simulink model "ap_12B_cocoSim_pp"  (Simulink 8.5)
settings: Solver=ode3  StartTime=0.0  StopTime=100  FixedStep=Ts  RelTol=1e-3
undefined symbols (not defined in the file): beaver_b, beaver_c, beaver_mass, beaver_S, Cl0, Cl_alpha2_dpt, Cl_beta, Cl_da, Cl_da_alpha, Cl_dr, Cl_p, Cl_r, Cm0, Cm_alpha, Cm_alpha2, Cm_beta2, Cm_de, Cm_df, Cm_dpt, Cm_q, Cm_r, Cn0, Cn_beta, Cn_beta3, Cn_da, Cn_dpt3, Cn_dr, Cn_p, Cn_q, Cn_r, Cx0, Cx_alpha, Cx_alpha2, Cx_alpha3, Cx_df, Cx_df_alpha, Cx_dpt, Cx_dpt2_alpha, Cx_dr, Cx_q, Cy0, Cy_beta, Cy_da, Cy_dr, Cy_dr_alpha, Cy_p, Cy_r, Cz0, Cz_alpha, Cz_alpha3, Cz_de, Cz_de_beta, Cz_df, Cz_df_alpha, Cz_dpt, Cz_q, d2r, fin_act_1, fin_act_2, fin_act_3 ... (+23)
libraries: simulink x12, aerolibtransform2 x9, aerolibutil x7, aerolibasang x7, aerolibadynsys x3, aerolib6dofsys x2, aerolib6dof2 x1
(part 1 of 3)
settings Model: Creator=elliocm  LastModifiedBy=Teme
settings DataIOCC: SignalLoggingSaveFormat=Dataset
settings DebuggingCC: SolverPrmCheckMsg=warning  FcnCallInpInsideContextMsg=EnableAllAsError
settings GRTTargetCC: CombineOutputUpdateFcns=on  GRTInterface=off

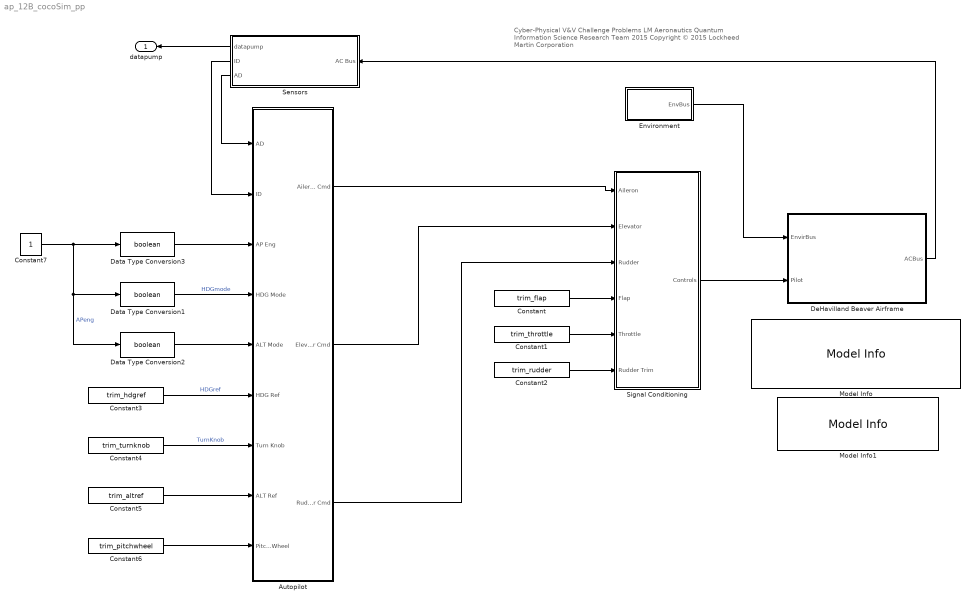
== system ap_12B_cocoSim_pp ==
  note: Cyber-Physical V&V Challenge Problems
      | LM Aeronautics Quantum Information Science Research Team 2015
      | Copyright © 2015 Lockheed Martin Corporation
  Autopilot : Subsystem
  Constant : Constant  Value=trim_flap
  Constant1 : Constant  Value=trim_throttle
  Constant2 : Constant  Value=trim_rudder
  Constant3 : Constant  Value=trim_hdgref
  Constant4 : Constant  Value=trim_turnknob
  Constant5 : Constant  Value=trim_altref
  Constant6 : Constant  Value=trim_pitchwheel
  Constant7 : Constant
  Data Type Conversion1 : DataTypeConversion  OutDataTypeStr=boolean
  Data Type Conversion2 : DataTypeConversion  OutDataTypeStr=boolean
  Data Type Conversion3 : DataTypeConversion  OutDataTypeStr=boolean
  DeHavilland Beaver Airframe : Subsystem
      mask Display: image(imread('asbbeaver.jpg'))
  Environment : Subsystem
  Model Info : simulink/Model-Wide Utilities/Model Info  BlockCM=None  Frame=on  DisplayStringWithTags=|  HorizontalTextAlignment=Center  LeftAlignmentValue=0.5  SourceBlockDiagram=ap_12B_cocoSim_pp  TagMaxNumber=20
      | DeHavilland Beaver model 
      | originally based on work created by
      | Marc Rauw for Delft University of Technology,  
      | http://www.dutchroll.com
      | and subsequently modified by the Mathworks
      | http://www.mathworks.com/matlabcentral/fileexchange/
  Model Info1 : simulink/Model-Wide Utilities/Model Info  BlockCM=None  Frame=on  DisplayStringWithTags=|  HorizontalTextAlignment=Left  LeftAlignmentValue=0.02  SourceBlockDiagram=ap_12B_cocoSim_pp  TagMaxNumber=20
      | FLIGHT CONTROL Demonstration
      | Author: %<LastModifiedBy>
      | Model Version: %<ModelVersion>
      | Date: %<LastModificationDate>
  Sensors : Subsystem
  Signal Conditioning : Subsystem
  datapump : Outport
  wires:
  Constant7/1 -> Data Type Conversion2/1, Data Type Conversion1/1, Data Type Conversion3/1  "APeng"
  Data Type Conversion1/1 -> Autopilot/4(HDG Mode)  "HDGmode"
  Data Type Conversion2/1 -> Autopilot/5(ALT Mode)
  Constant3/1 -> Autopilot/6(HDG Ref)  "HDGref"
  Constant4/1 -> Autopilot/7(Turn Knob)  "TurnKnob"
  Constant5/1 -> Autopilot/8(ALT Ref)
  Constant6/1 -> Autopilot/9(Pitch Wheel)
  Autopilot/1(Aileron Cmd) -> Signal Conditioning/1(Aileron)
  Autopilot/2(Elevator Cmd) -> Signal Conditioning/2(Elevator)
  Autopilot/3(Rudder Cmd) -> Signal Conditioning/3(Rudder)
  DeHavilland Beaver Airframe/1(ACBus) -> Sensors/1(AC Bus)
  Constant/1 -> Signal Conditioning/4(Flap)
  Constant1/1 -> Signal Conditioning/5(Throttle)
  Constant2/1 -> Signal Conditioning/6(Rudder Trim)
  Signal Conditioning/1(Controls) -> DeHavilland Beaver Airframe/2(Pilot)
  Environment/1(EnvBus) -> DeHavilland Beaver Airframe/1(EnvirBus)
  Sensors/3(AD) -> Autopilot/1(AD)
  Sensors/2(ID) -> Autopilot/2(ID)
  Data Type Conversion3/1 -> Autopilot/3(AP Eng)
  Sensors/1(datapump) -> datapump/1

== system ap_12B_cocoSim_pp/Autopilot ==
  note: Autopilot
  AD : Inport
  ID : Inport  Port=2
  AP Eng : Inport  Port=3  OutMin=0  OutMax=1  OutDataTypeStr=boolean  PortDimensions=1
  HDG Mode : Inport  Port=4  OutMin=0  OutMax=1  OutDataTypeStr=boolean  PortDimensions=1
  ALT Mode : Inport  Port=5  OutMin=0  OutMax=1  OutDataTypeStr=boolean  PortDimensions=1
  HDG Ref : Inport  Port=6  OutMin=-180  OutMax=180  OutDataTypeStr=double  PortDimensions=1
  Turn Knob : Inport  Port=7  OutMin=-45  OutMax=45  OutDataTypeStr=double  PortDimensions=1
  ALT Ref : Inport  Port=8  OutMin=0  OutMax=65000  OutDataTypeStr=double  PortDimensions=1
  Pitch Wheel : Inport  Port=9  OutMin=-30  OutMax=30  OutDataTypeStr=double  PortDimensions=1
  Bus Selector : BusSelector  OutputSignals=phi,psi,p,theta,q,r
  Bus Selector1 : BusSelector  OutputSignals=alt,altRate,airspeed
  Model Info : simulink/Model-Wide Utilities/Model Info  BlockCM=None  Frame=on  DisplayStringWithTags=|  HorizontalTextAlignment=Left  LeftAlignmentValue=0.02  SourceBlockDiagram=ap_12B_cocoSim_pp  TagMaxNumber=20
      | Autopilot
      | Author: %<LastModifiedBy>
      | Date: %<LastModificationDate>
      | Model Version: %<ModelVersion>
  Pitch_Autopilot : Subsystem
  Roll_Autopilot : Subsystem
  Yaw_damper : Subsystem
  Aileron Cmd : Outport  OutDataTypeStr=double  PortDimensions=1  SampleTime=[0.025000000000000001,0]
  Elevator Cmd : Outport  Port=2  OutDataTypeStr=double  PortDimensions=1  SampleTime=[0.025000000000000001,0]
  Rudder Cmd : Outport  Port=3  OutDataTypeStr=double  PortDimensions=1  SampleTime=[0.025000000000000001,0]
  wires:
  Roll_Autopilot/1(Ail Cmd) -> Aileron Cmd/1
  HDG Ref/1 -> Roll_Autopilot/7(HDG Ref)
  Bus Selector/6 -> Yaw_damper/2(R), Pitch_Autopilot/4(R)  "<r>"
  Bus Selector1/3 -> Yaw_damper/3(TAS), Roll_Autopilot/4(TAS), Pitch_Autopilot/7(TAS)  "<airspeed>"
  HDG Mode/1 -> Roll_Autopilot/6(HDG Mode)
  Pitch_Autopilot/1(Elv Cmd) -> Elevator Cmd/1
  ALT Mode/1 -> Pitch_Autopilot/9(ALT Mode)
  ALT Ref/1 -> Pitch_Autopilot/10(Alt Ref)
  Pitch Wheel/1 -> Pitch_Autopilot/11("Pitch Wheel ")
  Bus Selector1/1 -> Pitch_Autopilot/5(Alt)  "<alt>"
  Yaw_damper/1(Rud Cmd) -> Rudder Cmd/1
  AP Eng/1 -> Yaw_damper/4(AP Eng), Roll_Autopilot/5(AP Eng), Pitch_Autopilot/8(AP Eng1)
  Bus Selector/3 -> Roll_Autopilot/3(p)  "<p>"
  Turn Knob/1 -> Roll_Autopilot/8(Turn Knob)
  Bus Selector/1 -> Pitch_Autopilot/1(Phi), Yaw_damper/1(Phi), Roll_Autopilot/1(Phi)  "<phi>"
  Bus Selector/2 -> Roll_Autopilot/2(Psi)  "<psi>"
  Bus Selector/5 -> Pitch_Autopilot/3(Q)  "<q>"
  Bus Selector/4 -> Pitch_Autopilot/2(Theta)  "<theta>"
  ID/1 -> Bus Selector/1
  AD/1 -> Bus Selector1/1
  Bus Selector1/2 -> Pitch_Autopilot/6(Alt Rate)  "<altRate>"

== system ap_12B_cocoSim_pp/DeHavilland Beaver Airframe ==
  note: DeHavilland Beaver Airframe
  EnvirBus : Inport
  Pilot : Inport  Port=2
  Aircraft Dynamics : Subsystem
  Calculate Parameters : Subsystem
  ACBus : Outport
  wires:
  Pilot/1 -> Aircraft Dynamics/1(Pilot)
  Aircraft Dynamics/1(AC Bus) -> ACBus/1, Calculate Parameters/2(ACBus)
  EnvirBus/1 -> Aircraft Dynamics/2(EnvirBus), Calculate Parameters/1(EnvirBus)
  Calculate Parameters/1(FltParams) -> Aircraft Dynamics/3(FltParams)

== system ap_12B_cocoSim_pp/Environment ==
  note: Environment
  Bus Creator : BusCreator  Inputs=3
  Bus Creator1 : BusCreator  Inputs=2
  Mux : Mux  Inputs=3
  Mux1 : Mux  Inputs=3
  g_mps2 : Constant  Value=9.799
  rho_kgpm3 : Constant  Value=0.9862
  wind_mps : Constant  Value=0
  EnvBus : Outport
  wires:
  g_mps2/1 -> Bus Creator/1  "g"
  Mux1/1 -> Bus Creator1/2  "pqr_wind"
  Mux/1 -> Bus Creator1/1  "uvw_wind"
  Bus Creator1/1 -> Bus Creator/3  "Vwind"
  Bus Creator/1 -> EnvBus/1
  rho_kgpm3/1 -> Bus Creator/2  "rho"
  wind_mps/1 -> Mux1/3, Mux1/2, Mux1/1, Mux/3, Mux/2, Mux/1

== system ap_12B_cocoSim_pp/Sensors ==
  AC Bus : Inport
  Air Data Sensor : Subsystem
  Bus Creator : BusCreator  Inputs=6
  Bus Creator1 : BusCreator  Inputs=5
  Bus Creator2 : BusCreator  Inputs=2
  Display : Display
  Display1 : Display
  Inertial Data Sensor : Subsystem
  Scope : Scope  NumInputPorts=5
      settings: YMin=-125~-3.5~-1.75~65~2000  YMax=125~3.5~1.75~150~7500  SaveName=ScopeData11
  Scope1 : Scope  NumInputPorts=6
      settings: YMin=-5~-5~-5~-5~-5~-5  YMax=5~5~5~5~5~5  SaveName=ScopeData12
  datapump : Outport
  ID : Outport  Port=2
  AD : Outport  Port=3
  wires:
  AC Bus/1 -> Air Data Sensor/1(AC Bus), Inertial Data Sensor/1(AC Bus)
  Inertial Data Sensor/3(psi) -> Scope1/3, Bus Creator/3  "psi"
  Inertial Data Sensor/2(theta) -> Scope1/2, Bus Creator/2  "theta"
  Inertial Data Sensor/4(p) -> Scope1/4, Bus Creator/4  "p"
  Inertial Data Sensor/1(phi) -> Scope1/1, Bus Creator/1
  Inertial Data Sensor/5(q) -> Scope1/5, Bus Creator/5  "q"
  Inertial Data Sensor/6(r) -> Scope1/6, Bus Creator/6  "r"
  Bus Creator/1 -> Bus Creator2/1, Display/1, ID/1  "ID"
  Air Data Sensor/1(altRate) -> Scope/1, Bus Creator1/1  "altRate"
  Air Data Sensor/2(alpha) -> Scope/2, Bus Creator1/2  "alpha"
  Air Data Sensor/3(beta) -> Scope/3, Bus Creator1/3  "beta"
  Air Data Sensor/4(airspeed) -> Scope/4, Bus Creator1/4  "airspeed"
  Air Data Sensor/5(alt) -> Scope/5, Bus Creator1/5  "alt"
  Bus Creator1/1 -> Bus Creator2/2, Display1/1, AD/1  "AD"
  Bus Creator2/1 -> datapump/1

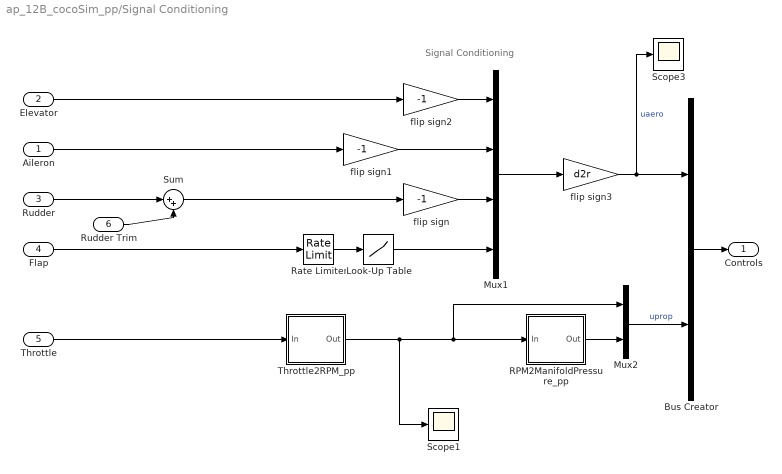
== system ap_12B_cocoSim_pp/Signal Conditioning ==
  note: Signal Conditioning
  Aileron : Inport
  Elevator : Inport  Port=2
  Rudder : Inport  Port=3
  Flap : Inport  Port=4
  Throttle : Inport  Port=5
  Rudder Trim : Inport  Port=6
  Bus Creator : BusCreator  Inputs=2
  Look-Up Table : Lookup  InputValues=[0:3]  Table=[0 4 10 20]  SaturateOnIntegerOverflow=on
  Mux1 : Mux
  Mux2 : Mux  Inputs=2
  RPM2ManifoldPressure_pp : Subsystem  TreatAsAtomicUnit=on
  Rate Limiter : RateLimiter  RisingSlewLimit=0.5  FallingSlewLimit=-0.5
  Scope1 : Scope
      settings: SaveName=ScopeData7
  Scope3 : Scope
      settings: SaveName=ScopeData6
  Sum : Sum  Inputs=|++
  Throttle2RPM_pp : Subsystem  TreatAsAtomicUnit=on
  flip sign : Gain  Gain=-1  SaturateOnIntegerOverflow=on  OutDataTypeStr=Inherit: Same as input  ParamDataTypeStr=Inherit: Same as input
  flip sign1 : Gain  Gain=-1  SaturateOnIntegerOverflow=on  OutDataTypeStr=Inherit: Same as input  ParamDataTypeStr=Inherit: Same as input
  flip sign2 : Gain  Gain=-1  SaturateOnIntegerOverflow=on  OutDataTypeStr=Inherit: Same as input  ParamDataTypeStr=Inherit: Same as input
  flip sign3 : Gain  Gain=d2r  SaturateOnIntegerOverflow=on  OutDataTypeStr=Inherit: Same as input  ParamDataTypeStr=Inherit: Same as input
  Controls : Outport
  wires:
  Bus Creator/1 -> Controls/1
  Throttle/1 -> Throttle2RPM_pp/1(In)
  Sum/1 -> flip sign/1
  Aileron/1 -> flip sign1/1
  Elevator/1 -> flip sign2/1
  flip sign2/1 -> Mux1/1
  flip sign1/1 -> Mux1/2
  Throttle2RPM_pp/1(Out) -> Scope1/1, RPM2ManifoldPressure_pp/1(In), Mux2/1
  flip sign/1 -> Mux1/3
  Mux2/1 -> Bus Creator/2  "uprop"
  RPM2ManifoldPressure_pp/1(Out) -> Mux2/2
  flip sign3/1 -> Scope3/1, Bus Creator/1  "uaero"
  Mux1/1 -> flip sign3/1
  Look-Up Table/1 -> Mux1/4
  Rate Limiter/1 -> Look-Up Table/1
  Rudder/1 -> Sum/1
  Rudder Trim/1 -> Sum/2
  Flap/1 -> Rate Limiter/1

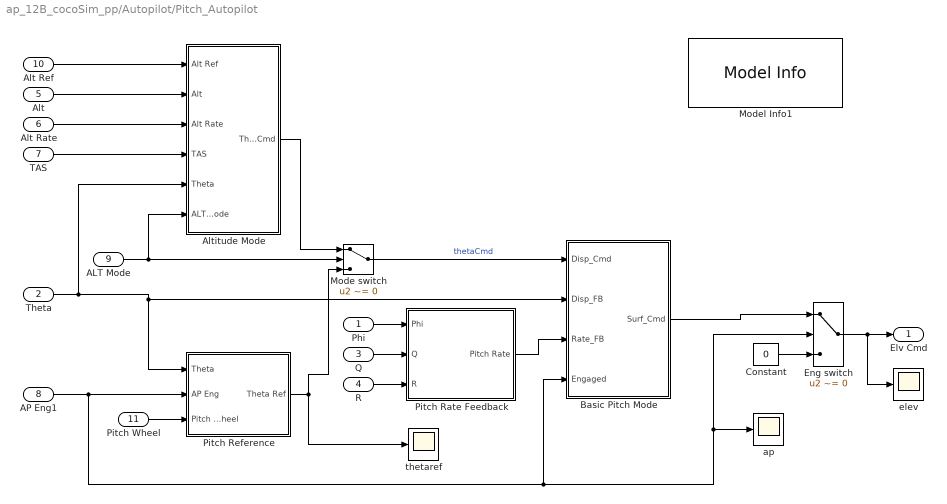
== system ap_12B_cocoSim_pp/Autopilot/Pitch_Autopilot ==
  Phi : Inport  OutDataTypeStr=double  PortDimensions=1  SampleTime=1/40  Interpolate=off
  Theta : Inport  Port=2  OutDataTypeStr=double  PortDimensions=1  SampleTime=1/40  Interpolate=off
  Q : Inport  Port=3  OutDataTypeStr=double  PortDimensions=1  SampleTime=1/40  Interpolate=off
  R : Inport  Port=4  OutDataTypeStr=double  PortDimensions=1  SampleTime=1/40  Interpolate=off
  Alt : Inport  Port=5  OutDataTypeStr=double  PortDimensions=1  SampleTime=1/40  Interpolate=off
  Alt Rate : Inport  Port=6  OutDataTypeStr=double  PortDimensions=1  SampleTime=1/40  Interpolate=off
  TAS : Inport  Port=7  OutDataTypeStr=double  PortDimensions=1  SampleTime=1/40  Interpolate=off
  AP Eng1 : Inport  Port=8  OutDataTypeStr=boolean  PortDimensions=1  SampleTime=1/40  Interpolate=off
  ALT Mode : Inport  Port=9  OutDataTypeStr=boolean  PortDimensions=1  SampleTime=1/40  Interpolate=off
  Alt Ref : Inport  Port=10  OutDataTypeStr=double  PortDimensions=1  SampleTime=1/40  Interpolate=off
  "Pitch Wheel " : Inport  Port=11  OutDataTypeStr=double  PortDimensions=1  SampleTime=1/40  Interpolate=off
  Altitude Mode : Subsystem
  Basic Pitch Mode : Subsystem
  Constant : Constant  Value=0  OutDataTypeStr=double
  Eng switch : Switch  Criteria=u2 ~= 0
  Mode switch : Switch  Criteria=u2 ~= 0
  Model Info1 : simulink/Model-Wide Utilities/Model Info  BlockCM=None  Frame=on  DisplayStringWithTags=|  HorizontalTextAlignment=Left  LeftAlignmentValue=0.02  SourceBlockDiagram=ap_12B_cocoSim_pp  TagMaxNumber=20
      | Pitch Autopilot
      | Author: %<LastModifiedBy>
      | Date: %<LastModificationDate>
      | Model Version: %<ModelVersion>
  Pitch Rate Feedback : Subsystem  TreatAsAtomicUnit=on
      settings: RTWSystemCode=Inline
  Pitch Reference : Subsystem  TreatAsAtomicUnit=on
      settings: RTWSystemCode=Inline
  ap : Scope
      settings: SaveName=ScopeData29
  elev : Scope
      settings: SaveName=ScopeData33
  thetaref : Scope
      settings: SaveName=ScopeData37
  Elv Cmd : Outport  OutDataTypeStr=double  PortDimensions=1  SampleTime=1/40
  wires:
  "Pitch Wheel "/1 -> Pitch Reference/3(Pitch Wheel)
  Pitch Rate Feedback/1(Pitch Rate) -> Basic Pitch Mode/3(Rate_FB)
  Alt Ref/1 -> Altitude Mode/1(Alt Ref)
  Theta/1 -> Altitude Mode/5(Theta), Pitch Reference/1(Theta), Basic Pitch Mode/2("Disp_FB ")
  Q/1 -> Pitch Rate Feedback/2(Q)
  Eng switch/1 -> elev/1, Elv Cmd/1
  Constant/1 -> Eng switch/3
  Phi/1 -> Pitch Rate Feedback/1(Phi)
  R/1 -> Pitch Rate Feedback/3(R)
  TAS/1 -> Altitude Mode/4(TAS)
  Pitch Reference/1(Theta Ref) -> thetaref/1, Mode switch/3
  Alt/1 -> Altitude Mode/2(Alt)
  Alt Rate/1 -> Altitude Mode/3(Alt Rate)
  Mode switch/1 -> Basic Pitch Mode/1(Disp_Cmd)  "thetaCmd"
  ALT Mode/1 -> Altitude Mode/6(ALT Mode), Mode switch/2
  Altitude Mode/1(Theta Cmd) -> Mode switch/1
  AP Eng1/1 -> Eng switch/2, ap/1, Basic Pitch Mode/4(Engaged), Pitch Reference/2(AP Eng)
  Basic Pitch Mode/1(Surf_Cmd) -> Eng switch/1

== system ap_12B_cocoSim_pp/Autopilot/Roll_Autopilot ==
  Phi : Inport  RequirementInfo={'other' 'do178b_autopilot_requirements.docx' '@Simulink_requirement_item_3' 'true' '1.3. Roll Hold Reference' ' ' ; 'other' 'do178b_autopilot_requirements.docx' '@Simulink_requirement_item_4' 'true' '1.4. Roll Performance' '' } %GIDa_bd230888_8e4f_4651_af95_bb052af88046  OutMin=-180  OutMax=180  OutDataTypeStr=double  PortDimensions=1  SampleTime=1/40  Interpolate=off
  Psi : Inport  RequirementInfo={'other' 'do178b_autopilot_requirements.docx' '@Simulink_requirement_item_10' 'true' '1.10. Heading Performance' '' } %GIDa_dd31966d_985c_45f4_accd_9bdc5dfb2899  Port=2  OutMin=-180  OutMax=180  OutDataTypeStr=double  PortDimensions=1  SampleTime=1/40  Interpolate=off
  p : Inport  RequirementInfo={'other' 'do178b_autopilot_requirements.docx' '@Simulink_requirement_item_4' 'true' '1.4. Roll Performance' '' } %GIDa_df9fbc51_a2ae_43d6_98fc_cabd7d0ca57e  Port=3  OutMin=-180  OutMax=180  OutDataTypeStr=double  PortDimensions=1  Interpolate=off
  TAS : Inport  RequirementInfo={'other' 'do178b_autopilot_requirements.docx' '@Simulink_requirement_item_10' 'true' '1.10. Heading Performance' '' } %GIDa_635b1e96_333c_4ec3_a8eb_fd034fb3c326  Port=4  OutMin=0  OutMax=1000  OutDataTypeStr=double  PortDimensions=1  SampleTime=1/40  Interpolate=off
  AP Eng : Inport  RequirementInfo={'other' 'do178b_autopilot_requirements.docx' '@Simulink_requirement_item_1' 'true' '1.1. Roll Autopilot Engage Control' ' ' ; 'other' 'do178b_autopilot_requirements.docx' '@Simulink_requirement_item_3' 'true' '1.3. Roll Hold Reference' ' ' ; 'other' 'do178b_autopilot_requirements.docx' '@Simulink_requirement_item_4' 'true' '1.4. Roll Performance' '' } %GIDa_32c51ab2_ea73_4f85_bfd4_20a740fc7588  Port=5  OutDataTypeStr=boolean  PortDimensions=1  SampleTime=1/40  Interpolate=off
  HDG Mode : Inport  RequirementInfo={'other' 'do178b_autopilot_requirements.docx' '@Simulink_requirement_item_2' 'true' '1.2. Roll Hold Mode' ' ' ; 'other' 'do178b_autopilot_requirements.docx' '@Simulink_requirement_item_8' 'true' '1.8. Heading Hold Mode' '' } %GIDa_2622cebb_32cd_44ec_b3f0_415d7d3b06da  Port=6  OutDataTypeStr=boolean  PortDimensions=1  SampleTime=1/40  Interpolate=off
  HDG Ref : Inport  RequirementInfo={'other' 'do178b_autopilot_requirements.docx' '@Simulink_requirement_item_9' 'true' '1.9. Heading Hold Reference' ' ' ; 'other' 'do178b_autopilot_requirements.docx' '@Simulink_requirement_item_10' 'true' '1.10. Heading Performance' '' } %GIDa_1720625b_9837_4e8c_b101_844eceaa1bed  Port=7  OutMin=-180  OutMax=180  OutDataTypeStr=double  PortDimensions=1  SampleTime=1/40  Interpolate=off
  Turn Knob : Inport  RequirementInfo={'other' 'do178b_autopilot_requirements.docx' '@Simulink_requirement_item_3' 'true' '1.3. Roll Hold Reference' '' } %GIDa_9853f841_f607_4644_995f_a277bee0f0d4  Port=8  OutMin=-45  OutMax=45  OutDataTypeStr=double  PortDimensions=1  SampleTime=1/40  Interpolate=off
  Basic Roll Mode : Subsystem
  Eng switch : Switch  RequirementInfo={'other' 'do178b_autopilot_requirements.docx' '' 'true' '1.1. Roll Autopilot Engage Control' ' ' } %GIDa_48ca80c0_8a95_4669_9a3a_89e9ba2b13bd  Criteria=u2 ~= 0
  Heading Mode : Subsystem
  Mode switch : Switch  RequirementInfo={'other' 'do178b_autopilot_requirements.docx' '@Simulink_requirement_item_2' 'true' '1.2. Roll Hold Mode' ' ' ; 'other' 'do178b_autopilot_requirements.docx' '@Simulink_requirement_item_4' 'true' '1.4. Roll Performance' ' ' ; 'other' 'do178b_autopilot_requirements.docx' '@Simulink_requirement_item_8' 'true' '1.8. Heading Hold Mode' ' ' ; 'other' 'do178b_autopilot_requirements.docx' '@Simulink_requirement_item_10' 'true' '1.10. Heading Performance' '' } %GIDa_7ff7f3f6_daae_4da2_99fc_89be4661dc9b  Criteria=u2 ~= 0
  Model Info : simulink/Model-Wide Utilities/Model Info  RequirementInfo={} %GIDa_8a06d8a3_adc0_4540_b134_32bcff30f9aa  BlockCM=None  Frame=on  DisplayStringWithTags=|  HorizontalTextAlignment=Left  LeftAlignmentValue=0.02  SourceBlockDiagram=ap_12B_cocoSim_pp  TagMaxNumber=20
      | Roll Autopilot
      | Author: %<LastModifiedBy>
      | Model Version: %<ModelVersion>
      | Date: %<LastModificationDate>
  Roll Reference : Subsystem  RequirementInfo={'other' 'do178b_autopilot_requirements.docx' '@Simulink_requirement_item_3' 'true' '1.3. Roll Hold Reference' '' } %GIDa_54b8aa08_ab27_4ed0_a6e8_f116b5006373  TreatAsAtomicUnit=on
      settings: RTWSystemCode=Inline
  zero : Constant  RequirementInfo={'other' 'do178b_autopilot_requirements.docx' '' 'true' '1.1. Roll Autopilot Engage Control' '' } %GIDa_447f47c4_0c8a_430f_82c0_d7755d441746  Value=0  OutDataTypeStr=double
  Ail Cmd : Outport  RequirementInfo={'other' 'do178b_autopilot_requirements.docx' '' 'true' '1.1. Roll Autopilot Engage Control' ' ' } %GIDa_ea4f82f9_e42f_4b8f_8523_427f9e113761  OutDataTypeStr=double  PortDimensions=1  SampleTime=1/40
  wires:
  HDG Ref/1 -> Heading Mode/1(Psi Ref)
  Heading Mode/1(Phi Cmd) -> Mode switch/1
  Basic Roll Mode/1(Surf_Cmd) -> Eng switch/1
  Mode switch/1 -> Basic Roll Mode/1(Disp_Cmd)  "phiCmd"
  Eng switch/1 -> Ail Cmd/1
  AP Eng/1 -> Roll Reference/2(AP eng), Basic Roll Mode/4(Engaged), Eng switch/2
  TAS/1 -> Heading Mode/3(TAS)
  HDG Mode/1 -> Mode switch/2
  Roll Reference/1(Phi Ref) -> Mode switch/3
  Turn Knob/1 -> Roll Reference/3(Turn Knob)
  zero/1 -> Eng switch/3
  p/1 -> Basic Roll Mode/3(Rate_FB)
  Phi/1 -> Basic Roll Mode/2("Disp_FB "), Roll Reference/1(Phi)
  Psi/1 -> Heading Mode/2(Psi)

== system ap_12B_cocoSim_pp/Autopilot/Yaw_damper ==
  Phi : Inport  OutDataTypeStr=double  PortDimensions=1  SampleTime=1/40  Interpolate=off
  R : Inport  Port=2  OutDataTypeStr=double  PortDimensions=1  SampleTime=1/40  Interpolate=off
  TAS : Inport  Port=3  OutDataTypeStr=double  PortDimensions=1  SampleTime=1/40  Interpolate=off
  AP Eng : Inport  Port=4  OutDataTypeStr=boolean  PortDimensions=1  SampleTime=1/40  Interpolate=off
  Basic Yaw Damper : Subsystem  TreatAsAtomicUnit=on
      settings: RTWSystemCode=Inline
  Constant : Constant  Value=0  OutDataTypeStr=double
  Eng switch : Switch  Criteria=u2 ~= 0
  Model Info1 : simulink/Model-Wide Utilities/Model Info  BlockCM=None  Frame=on  DisplayStringWithTags=|  HorizontalTextAlignment=Left  LeftAlignmentValue=0.02  SourceBlockDiagram=ap_12B_cocoSim_pp  TagMaxNumber=20
      | Yaw Damper
      | Author: %<LastModifiedBy>
      | Version: %<ModelVersion>
      | Date: %<LastModificationDate>
  Rud Cmd : Outport  OutDataTypeStr=double  PortDimensions=1  SampleTime=1/40
  wires:
  Phi/1 -> Basic Yaw Damper/1("Phi ")
  R/1 -> Basic Yaw Damper/2(R)
  Constant/1 -> Eng switch/3
  TAS/1 -> Basic Yaw Damper/3(TAS)
  Basic Yaw Damper/1(Rud Cmd) -> Eng switch/1
  Eng switch/1 -> Rud Cmd/1
  AP Eng/1 -> Eng switch/2

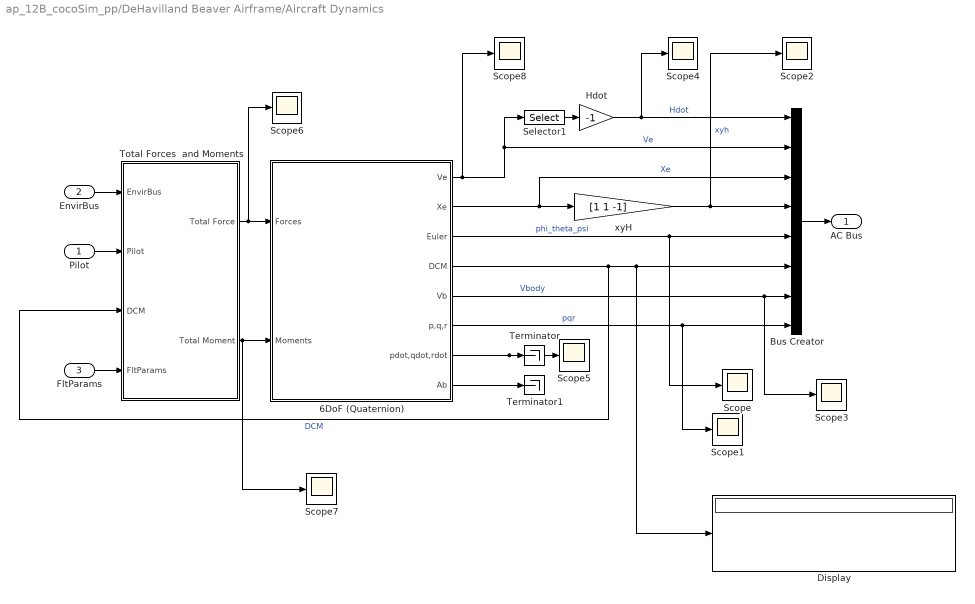
== system ap_12B_cocoSim_pp/DeHavilland Beaver Airframe/Aircraft Dynamics ==
  Pilot : Inport
  EnvirBus : Inport  Port=2
  FltParams : Inport  Port=3
  6DoF (Quaternion) : Subsystem
  Bus Creator : BusCreator  Inputs=8
  Display : Display
  Hdot : Gain  Gain=-1  SaturateOnIntegerOverflow=on  OutDataTypeStr=Inherit: Same as input  ParamDataTypeStr=Inherit: Same as input
  Scope{,1..8} (9 alike) : Scope
      Scope2 settings: SaveName=ScopeData2
      Scope3 settings: SaveName=ScopeData3
      Scope4 settings: SaveName=ScopeData5
      Scope5 settings: SaveName=ScopeData10
      Scope6 settings: SaveName=ScopeData20
      Scope7 settings: SaveName=ScopeData21
      Scope8 settings: SaveName=ScopeData23
  Selector1 : Selector  InputPortWidth=3  Indices=[3]
  Terminator : Terminator
  Terminator1 : Terminator
  Total Forces  and Moments : Subsystem
  xyH : Gain  Gain=[1 1 -1]  SaturateOnIntegerOverflow=on  OutDataTypeStr=Inherit: Same as input  ParamDataTypeStr=Inherit: Same as input
  AC Bus : Outport
  wires:
  6DoF (Quaternion)/4(DCM) -> Display/1, Bus Creator/6, Total Forces  and Moments/3(DCM)  "DCM"
  6DoF (Quaternion)/3(Euler) -> Scope/1, Bus Creator/5  "phi_theta_psi"
  6DoF (Quaternion)/2(Xe) -> xyH/1, Bus Creator/3  "Xe"
  6DoF (Quaternion)/5(Vb) -> Scope3/1, Bus Creator/7  "Vbody"
  6DoF (Quaternion)/7(pdot,qdot,rdot) -> Scope5/1, Terminator/1
  6DoF (Quaternion)/1(Ve) -> Scope8/1, Selector1/1, Bus Creator/2  "Ve"
  Pilot/1 -> Total Forces  and Moments/2(Pilot)
  Selector1/1 -> Hdot/1
  Total Forces  and Moments/1(Total Force) -> Scope6/1, 6DoF (Quaternion)/1(Forces)
  Total Forces  and Moments/2(Total Moment) -> Scope7/1, 6DoF (Quaternion)/2(Moments)
  xyH/1 -> Scope2/1, Bus Creator/4  "xyh"
  Hdot/1 -> Scope4/1, Bus Creator/1  "Hdot"
  6DoF (Quaternion)/8(Ab) -> Terminator1/1
  Bus Creator/1 -> AC Bus/1
  EnvirBus/1 -> Total Forces  and Moments/1(EnvirBus)
  6DoF (Quaternion)/6(p,q,r) -> Scope1/1, Bus Creator/8  "pqr"
  FltParams/1 -> Total Forces  and Moments/4(FltParams)

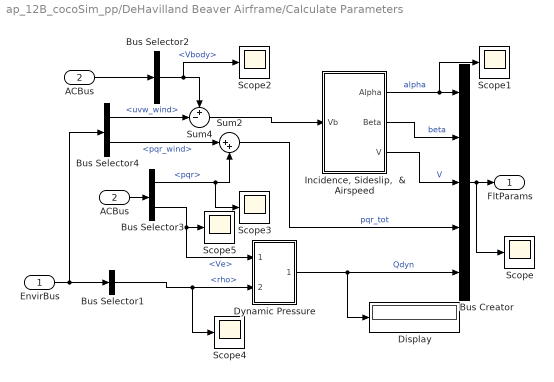
== system ap_12B_cocoSim_pp/DeHavilland Beaver Airframe/Calculate Parameters ==
  EnvirBus : Inport
  ACBus : Inport  Port=2
  " Incidence, Sideslip,  & Airspeed" : Subsystem
  "ACBus " : InportShadow  Port=2
  Bus Creator : BusCreator  Inputs=5
  Bus Selector1 : BusSelector  OutputSignals=rho
  Bus Selector2 : BusSelector  OutputSignals=Vbody
  Bus Selector3 : BusSelector  OutputSignals=pqr,Ve
  Bus Selector4 : BusSelector  OutputSignals=Vwind.uvw_wind,Vwind.pqr_wind
  Display : Display
  Dynamic Pressure : Subsystem
  Scope{,1..5} (6 alike) : Scope
      Scope settings: SaveName=ScopeData14
      Scope1 settings: SaveName=ScopeData15
      Scope2 settings: SaveName=ScopeData16
      Scope3 settings: SaveName=ScopeData17
      Scope4 settings: SaveName=ScopeData18
      Scope5 settings: SaveName=ScopeData19
  Sum2 : Sum  Inputs=|++  SaturateOnIntegerOverflow=on  InputSameDT=on  OutDataTypeStr=Inherit: Same as first input
  Sum4 : Sum  Inputs=+-|  SaturateOnIntegerOverflow=on  InputSameDT=on  OutDataTypeStr=Inherit: Same as first input
  FltParams : Outport
  wires:
  "ACBus "/1 -> Bus Selector2/1
  Bus Creator/1 -> Scope/1, FltParams/1
  Bus Selector3/1 -> Scope3/1, Sum2/2  "<pqr>"
  ACBus/1 -> Bus Selector3/1
  Bus Selector1/1 -> Scope4/1, Dynamic Pressure/2(Air Density)  "<rho>"
  EnvirBus/1 -> Bus Selector1/1, Bus Selector4/1
  Dynamic Pressure/1(qbar) -> Display/1, Bus Creator/5  "Qdyn"
  Bus Selector3/2 -> Scope5/1, Dynamic Pressure/1(Velocity)  "<Ve>"
  Bus Selector4/2 -> Sum2/1  "<pqr_wind>"
  Sum4/1 -> " Incidence, Sideslip,  & Airspeed"/1(Vb)
  " Incidence, Sideslip,  & Airspeed"/1(Alpha) -> Scope1/1, Bus Creator/1  "alpha"
  " Incidence, Sideslip,  & Airspeed"/2(Beta) -> Bus Creator/2  "beta"
  " Incidence, Sideslip,  & Airspeed"/3(V) -> Bus Creator/3  "V"
  Bus Selector2/1 -> Scope2/1, Sum4/1  "<Vbody>"
  Bus Selector4/1 -> Sum4/2  "<uvw_wind>"
  Sum2/1 -> Bus Creator/4  "pqr_tot"

== system ap_12B_cocoSim_pp/Sensors/Air Data Sensor ==
  note: Air Data Sensor
  AC Bus : Inport
  " Incidence, Sideslip,  & Airspeed" : Subsystem
  Bus Selector1 : BusSelector  OutputSignals=Hdot,Vbody,xyh
  Constant1 : Constant  Value=trim_v
  Constant2 : Constant  Value=0.0
  Constant3 : Constant  Value=trim_altref
  Selector1 : Selector  InputPortWidth=3  Indices=[3]
  flip sign1 : Gain  Gain=m2ft  SaturateOnIntegerOverflow=on  OutDataTypeStr=Inherit: Same as input  ParamDataTypeStr=Inherit: Same as input
  flip sign2 : Gain  Gain=m2ft  SaturateOnIntegerOverflow=on  OutDataTypeStr=Inherit: Same as input  ParamDataTypeStr=Inherit: Same as input
  flip sign3 : Gain  Gain=m2ft  SaturateOnIntegerOverflow=on  OutDataTypeStr=Inherit: Same as input  ParamDataTypeStr=Inherit: Same as input
  ic1 : Subsystem
  ic2 : Subsystem
  ic3 : Subsystem
  altRate : Outport
  alpha : Outport  Port=2
  beta : Outport  Port=3
  airspeed : Outport  Port=4
  alt : Outport  Port=5
  wires:
  Bus Selector1/1 -> flip sign2/1  "<Hdot>"
  ic1/1(y) -> flip sign1/1
  ic3/1(y) -> altRate/1  "altRate"
  Bus Selector1/3 -> Selector1/1  "<xyh>"
  flip sign1/1 -> " Incidence, Sideslip,  & Airspeed"/1(Vb)  "Vfps"
  " Incidence, Sideslip,  & Airspeed"/1(Alpha) -> alpha/1  "alpha"
  Bus Selector1/2 -> ic1/1(u)  "<Vbody>"
  AC Bus/1 -> Bus Selector1/1
  " Incidence, Sideslip,  & Airspeed"/3(V) -> airspeed/1  "airspeed"
  flip sign2/1 -> ic3/1(u)  "Hdotfps"
  Constant2/1 -> ic3/2(ic)
  Constant1/1 -> ic1/2(ic)
  Selector1/1 -> flip sign3/1
  ic2/1(y) -> alt/1  "alt"
  flip sign3/1 -> ic2/1(u)  "alt"
  Constant3/1 -> ic2/2(ic)
  " Incidence, Sideslip,  & Airspeed"/2(Beta) -> beta/1  "beta"

== system ap_12B_cocoSim_pp/Sensors/Inertial Data Sensor ==
  note: Inertial Data Sensor
  AC Bus : Inport
  Bus Selector : BusSelector  OutputSignals=phi_theta_psi,pqr
  Constant : Constant  Value=0.0
  Constant1 : Constant  Value=trim_hdg
  Constant2 : Constant  Value=0.0
  Constant3 : Constant  Value=trim_pitch
  Demux : Demux  Outputs=3
  Demux1 : Demux  Outputs=3
  flip sign1 : Gain  Gain=r2d  SaturateOnIntegerOverflow=on  OutDataTypeStr=Inherit: Same as input  ParamDataTypeStr=Inherit: Same as input
  flip sign3 : Gain  Gain=r2d  SaturateOnIntegerOverflow=on  OutDataTypeStr=Inherit: Same as input  ParamDataTypeStr=Inherit: Same as input
  ic : Subsystem
  ic1 : Subsystem
  ic2 : Subsystem
  ic3 : Subsystem
  phi : Outport
  theta : Outport  Port=2
  psi : Outport  Port=3
  p : Outport  Port=4
  q : Outport  Port=5
  r : Outport  Port=6
  wires:
  Demux/3 -> r/1  "r"
  Demux/1 -> p/1  "p"
  Demux1/3 -> ic1/1(u)
  flip sign3/1 -> Demux1/1
  Demux1/2 -> ic2/1(u)
  Demux1/1 -> ic3/1(u)
  Bus Selector/1 -> flip sign3/1  "<phi_theta_psi>"
  flip sign1/1 -> ic/1(u)
  Bus Selector/2 -> flip sign1/1  "<pqr>"
  AC Bus/1 -> Bus Selector/1
  Demux/2 -> q/1  "q"
  ic2/1(y) -> theta/1  "theta"
  ic3/1(y) -> phi/1  "phi"
  ic/1(y) -> Demux/1
  ic1/1(y) -> psi/1  "psi"
  Constant/1 -> ic/2(ic)
  Constant1/1 -> ic1/2(ic)
  Constant2/1 -> ic3/2(ic)
  Constant3/1 -> ic2/2(ic)

== system ap_12B_cocoSim_pp/Signal Conditioning/RPM2ManifoldPressure_pp ==
  In : Inport
  CompInfEq2 : RelationalOperator  Operator=<=  InputSameDT=on
  CompInfEq3 : RelationalOperator  Operator=<=  InputSameDT=on
  CompSup1 : RelationalOperator  InputSameDT=on
  CompSup2 : RelationalOperator  Operator=>  InputSameDT=on
  Data1 : Constant  Value=0
  Data2 : Constant  Value=22.5735
  Data3 : Constant  Value=26
  Idx1 : Constant  Value=0
  Idx2 : Constant  Value=1800
  Idx3 : Constant  Value=2300
  Interpolate1 : Subsystem
  Interpolate2 : Subsystem
  Product1 : Product  Inputs=***  SaturateOnIntegerOverflow=on  RndMeth=Zero  OutDataTypeStr=Inherit: Same as first input
  Product2 : Product  Inputs=***  SaturateOnIntegerOverflow=on  RndMeth=Zero  OutDataTypeStr=Inherit: Same as first input
  Sum : Sum  SaturateOnIntegerOverflow=on  InputSameDT=on  OutDataTypeStr=Inherit: Same as first input
  Out : Outport
  wires:
  In/1 -> Interpolate1/1(InportIn), CompSup1/1, Interpolate2/1(InportIn), CompSup2/1, CompInfEq2/1, CompInfEq3/1
  Idx1/1 -> Interpolate1/2(InportIdx1), CompSup1/2
  Data1/1 -> Interpolate1/4(InportData1)
  Interpolate1/1(Out) -> Product1/1
  CompSup1/1 -> Product1/2
  CompInfEq2/1 -> Product1/3
  Product1/1 -> Sum/1
  Idx2/1 -> Interpolate2/2(InportIdx1), CompSup2/2, Interpolate1/3(InportIdx2), CompInfEq2/2
  Data2/1 -> Interpolate2/4(InportData1), Interpolate1/5(InportData2)
  Interpolate2/1(Out) -> Product2/1
  CompSup2/1 -> Product2/2
  CompInfEq3/1 -> Product2/3
  Product2/1 -> Sum/2
  Idx3/1 -> Interpolate2/3(InportIdx2), CompInfEq3/2
  Data3/1 -> Interpolate2/5(InportData2)
  Sum/1 -> Out/1

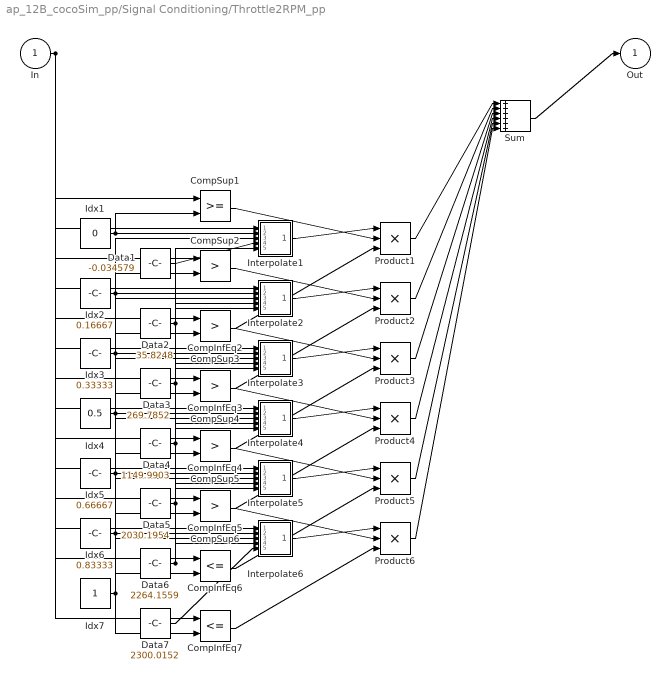
== system ap_12B_cocoSim_pp/Signal Conditioning/Throttle2RPM_pp ==
  In : Inport
  CompInfEq{2..7} (6 alike) : RelationalOperator  Operator=<=  InputSameDT=on
  CompSup1 : RelationalOperator  InputSameDT=on
  CompSup{2..6} (5 alike) : RelationalOperator  Operator=>  InputSameDT=on
  Data1 : Constant  Value=-0.034579
  Data2 : Constant  Value=35.8248
  Data3 : Constant  Value=269.7852
  Data4 : Constant  Value=1149.9903
  Data5 : Constant  Value=2030.1954
  Data6 : Constant  Value=2264.1559
  Data7 : Constant  Value=2300.0152
  Idx1 : Constant  Value=0
  Idx2 : Constant  Value=0.16667
  Idx3 : Constant  Value=0.33333
  Idx4 : Constant  Value=0.5
  Idx5 : Constant  Value=0.66667
  Idx6 : Constant  Value=0.83333
  Idx7 : Constant
  Interpolate1 : Subsystem
  Interpolate2 : Subsystem
  Interpolate3 : Subsystem
  Interpolate4 : Subsystem
  Interpolate5 : Subsystem
  Interpolate6 : Subsystem
  Product{1..6} (6 alike) : Product  Inputs=***  SaturateOnIntegerOverflow=on  RndMeth=Zero  OutDataTypeStr=Inherit: Same as first input
  Sum : Sum  Inputs=++++++  SaturateOnIntegerOverflow=on  InputSameDT=on  OutDataTypeStr=Inherit: Same as first input
  Out : Outport
  wires:
  In/1 -> Interpolate1/1(InportIn), CompSup1/1, Interpolate2/1(InportIn), CompSup2/1, CompInfEq2/1, Interpolate3/1(InportIn), CompSup3/1, CompInfEq3/1, Interpolate4/1(InportIn), CompSup4/1, CompInfEq4/1, Interpolate5/1(InportIn), CompSup5/1, CompInfEq5/1, Interpolate6/1(InportIn), CompSup6/1, CompInfEq6/1, CompInfEq7/1
  Idx1/1 -> Interpolate1/2(InportIdx1), CompSup1/2
  Data1/1 -> Interpolate1/4(InportData1)
  Interpolate1/1(Out) -> Product1/1
  CompSup1/1 -> Product1/2
  CompInfEq2/1 -> Product1/3
  Product1/1 -> Sum/1
  Idx2/1 -> Interpolate2/2(InportIdx1), CompSup2/2, Interpolate1/3(InportIdx2), CompInfEq2/2
  Data2/1 -> Interpolate2/4(InportData1), Interpolate1/5(InportData2)
  Interpolate2/1(Out) -> Product2/1
  CompSup2/1 -> Product2/2
  CompInfEq3/1 -> Product2/3
  Product2/1 -> Sum/2
  Idx3/1 -> Interpolate3/2(InportIdx1), CompSup3/2, Interpolate2/3(InportIdx2), CompInfEq3/2
  Data3/1 -> Interpolate3/4(InportData1), Interpolate2/5(InportData2)
  Interpolate3/1(Out) -> Product3/1
  CompSup3/1 -> Product3/2
  CompInfEq4/1 -> Product3/3
  Product3/1 -> Sum/3
  Idx4/1 -> Interpolate4/2(InportIdx1), CompSup4/2, Interpolate3/3(InportIdx2), CompInfEq4/2
  Data4/1 -> Interpolate4/4(InportData1), Interpolate3/5(InportData2)
  Interpolate4/1(Out) -> Product4/1
  CompSup4/1 -> Product4/2
  CompInfEq5/1 -> Product4/3
  Product4/1 -> Sum/4
  Idx5/1 -> Interpolate5/2(InportIdx1), CompSup5/2, Interpolate4/3(InportIdx2), CompInfEq5/2
  Data5/1 -> Interpolate5/4(InportData1), Interpolate4/5(InportData2)
  Interpolate5/1(Out) -> Product5/1
  CompSup5/1 -> Product5/2
  CompInfEq6/1 -> Product5/3
  Product5/1 -> Sum/5
  Idx6/1 -> Interpolate6/2(InportIdx1), CompSup6/2, Interpolate5/3(InportIdx2), CompInfEq6/2
  Data6/1 -> Interpolate6/4(InportData1), Interpolate5/5(InportData2)
  Interpolate6/1(Out) -> Product6/1
  CompSup6/1 -> Product6/2
  CompInfEq7/1 -> Product6/3
  Product6/1 -> Sum/6
  Idx7/1 -> Interpolate6/3(InportIdx2), CompInfEq7/2
  Data7/1 -> Interpolate6/5(InportData2)
  Sum/1 -> Out/1

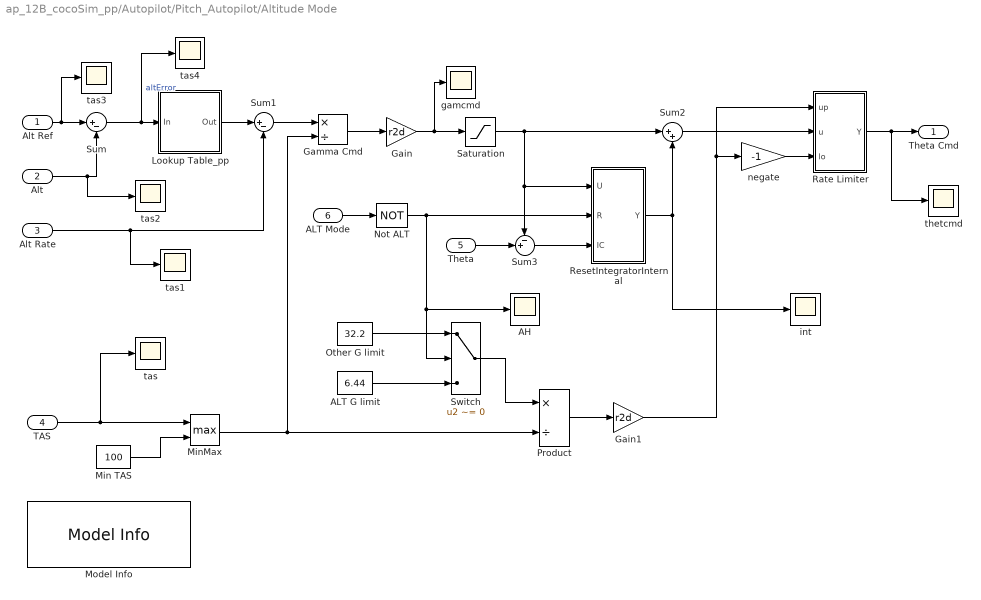
== system ap_12B_cocoSim_pp/Autopilot/Pitch_Autopilot/Altitude Mode ==
  Alt Ref : Inport  OutDataTypeStr=double  PortDimensions=1  SampleTime=1/40  Interpolate=off
  Alt : Inport  Port=2  OutDataTypeStr=double  PortDimensions=1  SampleTime=1/40  Interpolate=off
  Alt Rate : Inport  Port=3  OutDataTypeStr=double  PortDimensions=1  SampleTime=1/40  Interpolate=off
  TAS : Inport  Port=4  OutDataTypeStr=double  PortDimensions=1  SampleTime=1/40  Interpolate=off
  Theta : Inport  Port=5  OutDataTypeStr=double  PortDimensions=1  SampleTime=1/40  Interpolate=off
  ALT Mode : Inport  Port=6  OutDataTypeStr=boolean  PortDimensions=1  SampleTime=1/40  Interpolate=off
  AH : Scope
      settings: SaveName=ScopeData26
  ALT G limit : Constant  Value=6.44  OutDataTypeStr=double
  Gain : Gain  Gain=r2d
  Gain1 : Gain  Gain=r2d
  Gamma Cmd : Product  Inputs=*/  RndMeth=Zero
  Lookup Table_pp : Subsystem  TreatAsAtomicUnit=on
  Min TAS : Constant  Value=100  OutDataTypeStr=double
  MinMax : MinMax  Function=max  Inputs=2  InputSameDT=on
  Model Info : simulink/Model-Wide Utilities/Model Info  BlockCM=None  Frame=on  DisplayStringWithTags=|  HorizontalTextAlignment=Left  LeftAlignmentValue=0.02  SourceBlockDiagram=ap_12B_cocoSim_pp  TagMaxNumber=20
      | Altitude Mode
      | Author: %<LastModifiedBy>
      | Version: %<ModelVersion>
      | Date: %<LastModificationDate>
  Not ALT : Logic  Operator=NOT  IconShape=distinctive  AllPortsSameDT=off  OutDataTypeStr=boolean
  Other G limit : Constant  Value=32.2  OutDataTypeStr=double
  Product : Product  Inputs=*/  RndMeth=Zero
  Rate Limiter : Subsystem  mask(Rate Limiter Dynamic){}
      mask Display: plot([0.15 0.95],[.5 .5],[.5 .5],[0.05 0.95],0.05+0.9*[.2 .8],0.05+0.9*[0 1]);
  ResetIntegratorInternal : Subsystem
  Saturation : Saturate  UpperLimit=20  LowerLimit=-20
  Sum : Sum  Inputs=|+-
  Sum1 : Sum  Inputs=|+-
  Sum2 : Sum  Inputs=|++
  Sum3 : Sum  Inputs=-+|
  Switch : Switch  Criteria=u2 ~= 0
  gamcmd : Scope
      settings: SaveName=ScopeData31
  int : Scope
      settings: SaveName=ScopeData27
  negate : Gain  Gain=-1
  tas{,1..4} (5 alike) : Scope
      tas settings: SaveName=ScopeData28
      tas1 settings: SaveName=ScopeData38
      tas2 settings: SaveName=ScopeData39
      tas3 settings: SaveName=ScopeData40
      tas4 settings: SaveName=ScopeData41
  thetcmd : Scope
      settings: SaveName=ScopeData32
  Theta Cmd : Outport  OutDataTypeStr=double  PortDimensions=1  SampleTime=1/40
  wires:
  Other G limit/1 -> Switch/1
  Alt Ref/1 -> tas3/1, Sum/1
  Min TAS/1 -> MinMax/2
  Lookup Table_pp/1(Out) -> Sum1/1
  Rate Limiter/1(Y) -> thetcmd/1, Theta Cmd/1
  negate/1 -> Rate Limiter/3(lo)
  MinMax/1 -> Gamma Cmd/2, Product/2
  Product/1 -> Gain1/1
  Gain1/1 -> negate/1, Rate Limiter/1(up)
  Switch/1 -> Product/1
  ResetIntegratorInternal/1(Y) -> int/1, Sum2/2
  ALT G limit/1 -> Switch/3
  Sum2/1 -> Rate Limiter/2(u)
  Theta/1 -> Sum3/2
  Sum/1 -> tas4/1, Lookup Table_pp/1(In)  "altError"
  Saturation/1 -> Sum3/1, ResetIntegratorInternal/1(U), Sum2/1
  ALT Mode/1 -> Not ALT/1
  Gain/1 -> gamcmd/1, Saturation/1
  Alt/1 -> tas2/1, Sum/2
  Sum1/1 -> Gamma Cmd/1
  Alt Rate/1 -> tas1/1, Sum1/2
  Gamma Cmd/1 -> Gain/1
  Not ALT/1 -> AH/1, Switch/2, ResetIntegratorInternal/2(R)
  Sum3/1 -> ResetIntegratorInternal/3(IC)
  TAS/1 -> tas/1, MinMax/1

== system ap_12B_cocoSim_pp/Autopilot/Pitch_Autopilot/Basic Pitch Mode ==
  note: Attitude Control using displacement, rate and integral
  Disp_Cmd : Inport  RequirementInfo={} %GIDa_77e85a92_b978_4ff0_bd6d_d060380939d1  OutDataTypeStr=double  PortDimensions=1  SampleTime=1/40
  "Disp_FB " : Inport  RequirementInfo={} %GIDa_c41ff6c4_f4b0_4d96_9de3_c72981c15f52  Port=2  OutDataTypeStr=double  PortDimensions=1  SampleTime=1/40
  Rate_FB : Inport  RequirementInfo={} %GIDa_0e7c4d66_8c25_462f_8311_7596bc67b067  Port=3  OutDataTypeStr=double  PortDimensions=1  SampleTime=1/40
  Engaged : Inport  RequirementInfo={} %GIDa_c042823a_fe37_4d9c_975e_c69a7eabbe64  Port=4  OutDataTypeStr=boolean  PortDimensions=1  SampleTime=1/40
  Cmd Limit : Saturate  RequirementInfo={} %GIDa_5c035f2f_3105_4368_b211_79aac7692e87  UpperLimit=20  LowerLimit=-20
      settings: AttributesFormatString=%<LowerLimit> to %<UpperLimit> (deg)
  Disp Gain : Gain  RequirementInfo={} %GIDa_f8445782_a7ae_47ed_baa1_3a1981fda524  Gain=2.0
  Disp Limit : Saturate  RequirementInfo={} %GIDa_d1e93557_9df4_4290_b429_7e6cd706d281  UpperLimit=20  LowerLimit=-20
      settings: AttributesFormatString=%<LowerLimit> to %<UpperLimit> (deg)
  Int Gain : Gain  RequirementInfo={} %GIDa_8114a964_7a80_4a72_89cf_0ee832102f52  Gain=0.5
  Model Info : simulink/Model-Wide Utilities/Model Info  BlockCM=None  Frame=on  DisplayStringWithTags=|  HorizontalTextAlignment=Left  LeftAlignmentValue=0.02  SourceBlockDiagram=ap_12B_cocoSim_pp  TagMaxNumber=20
      | Attitude Controller
      | Author: %<LastModifiedBy>
      | Version: %<ModelVersion>
      | Date: %<LastModificationDate>
  Not engaged : Logic  RequirementInfo={} %GIDa_87ff32a2_d392_4896_a9d0_3aedb82f3c88  Operator=NOT  IconShape=distinctive  AllPortsSameDT=off  OutDataTypeStr=boolean
  Rate Gain : Gain  RequirementInfo={} %GIDa_b39ab451_9414_4b8d_b85e_7710fb1bd2ae  Gain=2.0
  Rate Limit : Saturate  RequirementInfo={} %GIDa_2af9c029_effe_4dc7_9b82_32fb64cde77c  UpperLimit=3  LowerLimit=-3
      settings: AttributesFormatString=%<LowerLimit> to %<UpperLimit> (deg/sec)
  ResetIntegratorInternal : Subsystem
  Sum : Sum  RequirementInfo={} %GIDa_4b6b4c1d_4d3f_4756_94a7_38849791cf07  Inputs=|+-
  Sum1 : Sum  RequirementInfo={} %GIDa_15a99a74_c04d_406f_862a_cb7e08471b6c  Inputs=|+-
  Sum2 : Sum  RequirementInfo={} %GIDa_ee7b0687_c2c3_44db_9f73_178d6ac0a19d  Inputs=++|
  att : Scope
      settings: SaveName=ScopeData30
  q : Scope
      settings: SaveName=ScopeData36
  thet : Scope
      settings: SaveName=ScopeData35
  Surf_Cmd : Outport  RequirementInfo={} %GIDa_36038573_f618_4da0_b90f_f44922f2e0fa  OutDataTypeStr=double  PortDimensions=1  SampleTime=1/40
  wires:
  Rate Limit/1 -> Sum1/1
  ResetIntegratorInternal/1(Y) -> Sum2/1, att/1
  Sum2/1 -> Cmd Limit/1
  Disp Limit/1 -> Sum/1
  Engaged/1 -> Not engaged/1
  Cmd Limit/1 -> Surf_Cmd/1
  Disp_Cmd/1 -> Disp Limit/1
  Rate_FB/1 -> q/1, Sum1/2
  Sum1/1 -> Rate Gain/1, Int Gain/1
  Sum/1 -> Disp Gain/1
  Disp Gain/1 -> Rate Limit/1
  Rate Gain/1 -> Sum2/2
  "Disp_FB "/1 -> thet/1, Sum/2
  Not engaged/1 -> ResetIntegratorInternal/2(R)
  Int Gain/1 -> ResetIntegratorInternal/1(U)

== system ap_12B_cocoSim_pp/Autopilot/Pitch_Autopilot/Pitch Rate Feedback ==
  note: Pitch Rate Computation
  Phi : Inport
  Q : Inport  Port=2
  R : Inport  Port=3
  Gain : Gain  Gain=d2r
  Product : Product  RndMeth=Zero
  Product1 : Product  RndMeth=Zero
  Sum3 : Sum  Inputs=|++
  cos : Trigonometry  Operator=cos  OutputSignalType=real
  q : Scope
      settings: SaveName=ScopeData34
  sin : Trigonometry  OutputSignalType=real
  Pitch Rate : Outport
  wires:
  Phi/1 -> Gain/1
  Product/1 -> Sum3/2
  sin/1 -> Product/1
  R/1 -> Product/2
  Gain/1 -> sin/1, cos/1
  Product1/1 -> Sum3/1
  cos/1 -> Product1/1
  Q/1 -> Product1/2
  Sum3/1 -> q/1, Pitch Rate/1

== system ap_12B_cocoSim_pp/Autopilot/Pitch_Autopilot/Pitch Reference ==
  note: Pitch Reference
  Theta : Inport
  AP Eng : Inport  Port=2
  Pitch Wheel : Inport  Port=3
  Not engaged : Logic  Operator=NOT  IconShape=distinctive  AllPortsSameDT=off  OutDataTypeStr=boolean
  Sum3 : Sum  Inputs=|++
  latch : Subsystem
  Theta Ref : Outport
  wires:
  Not engaged/1 -> latch/2(E)
  latch/1(y) -> Sum3/1
  Theta/1 -> latch/1(u)
  AP Eng/1 -> Not engaged/1
  Sum3/1 -> Theta Ref/1
  Pitch Wheel/1 -> Sum3/2

== system ap_12B_cocoSim_pp/Autopilot/Roll_Autopilot/Basic Roll Mode ==
  note: Attitude Control using displacement, rate and integral
  Disp_Cmd : Inport  RequirementInfo={} %GIDa_9cbdb2c4_acc8_4cf4_bad1_1cf810d967cc  OutDataTypeStr=double  PortDimensions=1
  "Disp_FB " : Inport  RequirementInfo={} %GIDa_570a039f_c58a_42ce_bf8c_8123d0436e35  Port=2  OutDataTypeStr=double  PortDimensions=1  SampleTime=1/40
  Rate_FB : Inport  RequirementInfo={} %GIDa_fa36bf04_50e7_4e7d_8666_47ec41fd0b8a  Port=3  OutDataTypeStr=double  PortDimensions=1  SampleTime=1/40
  Engaged : Inport  RequirementInfo={} %GIDa_c54d7bb2_857b_4779_8e1a_031b7c524bc4  Port=4  OutDataTypeStr=boolean  PortDimensions=1  SampleTime=1/40
  Cmd Limit : Saturate  RequirementInfo={} %GIDa_5206d30c_356d_4bfa_b564_1f4e9b4ba9a0  UpperLimit=15  LowerLimit=-15
      settings: AttributesFormatString=%<LowerLimit> to %<UpperLimit> (deg)
  Disp Gain : Gain  RequirementInfo={} %GIDa_85274674_3cfa_4c48_bfc7_c05fb49bd99e  Gain=1.0
  Disp Limit : Saturate  RequirementInfo={} %GIDa_5e5e7215_422b_4893_9c6c_b001fa1164f6  UpperLimit=30  LowerLimit=-30
      settings: AttributesFormatString=%<LowerLimit> to %<UpperLimit> (deg)
  Int Gain : Gain  RequirementInfo={} %GIDa_4d7f025a_88e2_4540_82a9_9d6514f74024  Gain=1.0
  Model Info : simulink/Model-Wide Utilities/Model Info  BlockCM=None  Frame=on  DisplayStringWithTags=|  HorizontalTextAlignment=Left  LeftAlignmentValue=0.02  SourceBlockDiagram=ap_12B_cocoSim_pp  TagMaxNumber=20
      | Attitude Controller
      | Author: %<LastModifiedBy>
      | Version: %<ModelVersion>
      | Date: %<LastModificationDate>
  Not engaged : Logic  RequirementInfo={} %GIDa_dd3a65b0_9756_4f26_bffe_ab1b7b4c647d  Operator=NOT  IconShape=distinctive  AllPortsSameDT=off  OutDataTypeStr=boolean
  Rate Gain : Gain  RequirementInfo={} %GIDa_116cf374_ddd9_4446_8b2c_40d18f1342df  Gain=3.0
  Rate Limit : Saturate  RequirementInfo={} %GIDa_2cf4c2c1_9f60_45b7_8b57_d0d2bd61766c  UpperLimit=6  LowerLimit=-6
      settings: AttributesFormatString=%<LowerLimit> to %<UpperLimit> (deg/sec)
  ResetIntegratorInternal : Subsystem
  Scope : Scope
      settings: SaveName=ScopeData8
  Scope1 : Scope
      settings: SaveName=ScopeData9
  Sum : Sum  RequirementInfo={} %GIDa_cbd80421_9144_4ab6_834f_65688c56bce3  Inputs=|+-
  Sum1 : Sum  RequirementInfo={} %GIDa_1afb3c0e_66db_4e97_838e_68e679123f7e  Inputs=|+-
  Sum2 : Sum  RequirementInfo={} %GIDa_07af5971_2786_425a_8b6c_f946ec91e63d  Inputs=++|
  Surf_Cmd : Outport  RequirementInfo={} %GIDa_d973f08f_89b0_4fd4_a3b3_c177716d5f15  OutDataTypeStr=double  PortDimensions=1  SampleTime=1/40
  wires:
  Engaged/1 -> Not engaged/1
  Disp_Cmd/1 -> Disp Limit/1
  Rate Limit/1 -> Sum1/1
  ResetIntegratorInternal/1(Y) -> Sum2/1, Scope/1
  Not engaged/1 -> ResetIntegratorInternal/2(R)
  Rate_FB/1 -> Sum1/2
  Sum1/1 -> Int Gain/1, Scope1/1, Rate Gain/1
  Cmd Limit/1 -> Surf_Cmd/1
  Rate Gain/1 -> Sum2/2
  Disp Gain/1 -> Rate Limit/1
  Sum/1 -> Disp Gain/1
  "Disp_FB "/1 -> Sum/2
  Disp Limit/1 -> Sum/1
  Sum2/1 -> Cmd Limit/1
  Int Gain/1 -> ResetIntegratorInternal/1(U)

== system ap_12B_cocoSim_pp/Autopilot/Roll_Autopilot/Heading Mode ==
  Psi Ref : Inport  RequirementInfo="{'other' 'do178b_autopilot_requirements.docx' '@Simulink_requirement_item_10' 'true' '1.10. Heading Performance    ' ' ' ; 'other' 'do178b_autopilot_requirements.docx' '@Simulink_requirement_item_9' 'true' '1.9. Heading Hold Reference' '' } %GIDa_a6cf1fd0_c062_4798_b010_50432035cd11"  OutDataTypeStr=double  PortDimensions=1  SampleTime=1/40  Interpolate=off
  Psi : Inport  RequirementInfo="{'other' 'do178b_autopilot_requirements.docx' '@Simulink_requirement_item_10' 'true' '1.10. Heading Performance     ' '' } %GIDa_eed26b28_0e5a_4ce0_9e15_5eb27554ca3d"  Port=2  OutDataTypeStr=double  PortDimensions=1  SampleTime=1/40  Interpolate=off
  TAS : Inport  RequirementInfo="{'other' 'do178b_autopilot_requirements.docx' '@Simulink_requirement_item_10' 'true' '1.10. Heading Performance        ' '' } %GIDa_cfb8053d_a47d_4eba_ae11_41b533f3512c"  Port=3  OutDataTypeStr=double  PortDimensions=1  SampleTime=1/40  Interpolate=off
  Disp Gain : Gain  RequirementInfo="{'other' 'do178b_autopilot_requirements.docx' '@Simulink_requirement_item_10' 'true' '1.10. Heading Performance       ' '' } %GIDa_84e8d514_db1c_497b_8580_46ac9c7c6ff1"  Gain=0.015
  Model Info : simulink/Model-Wide Utilities/Model Info  BlockCM=None  Frame=on  DisplayStringWithTags=|  HorizontalTextAlignment=Left  LeftAlignmentValue=0.02  SourceBlockDiagram=ap_12B_cocoSim_pp  TagMaxNumber=20
      | Heading Mode
      | Author: %<LastModifiedBy>
      | Version: %<ModelVersion>
      | Date: %<LastModificationDate>
  Product : Product  RequirementInfo="{'other' 'do178b_autopilot_requirements.docx' '@Simulink_requirement_item_10' 'true' '1.10. Heading Performance         ' '' } %GIDa_9e2d7d44_6434_4abd_b192_bfdb62210b9a"  RndMeth=Zero
  angle diff : Subsystem
  Phi Cmd : Outport  RequirementInfo="{'other' 'do178b_autopilot_requirements.docx' '@Simulink_requirement_item_10' 'true' '1.10. Heading Performance          ' '' } %GIDa_c1dcbb99_9d82_40a4_a35d_048de94d7014"  OutDataTypeStr=double  PortDimensions=1  SampleTime=1/40
  wires:
  Psi Ref/1 -> angle diff/1(plus)
  angle diff/1(diff) -> Disp Gain/1  "hdgError"
  TAS/1 -> Product/2
  Disp Gain/1 -> Product/1
  Psi/1 -> angle diff/2(minus)
  Product/1 -> Phi Cmd/1
